simulink model "converterstator"  (Simulink 7.3)
settings: Solver=ode23t  StartTime=0.0  StopTime=.9  RelTol=1e-3
libraries: powerlib x1
settings Model: Creator=lenovo  LastModifiedBy=lenovo

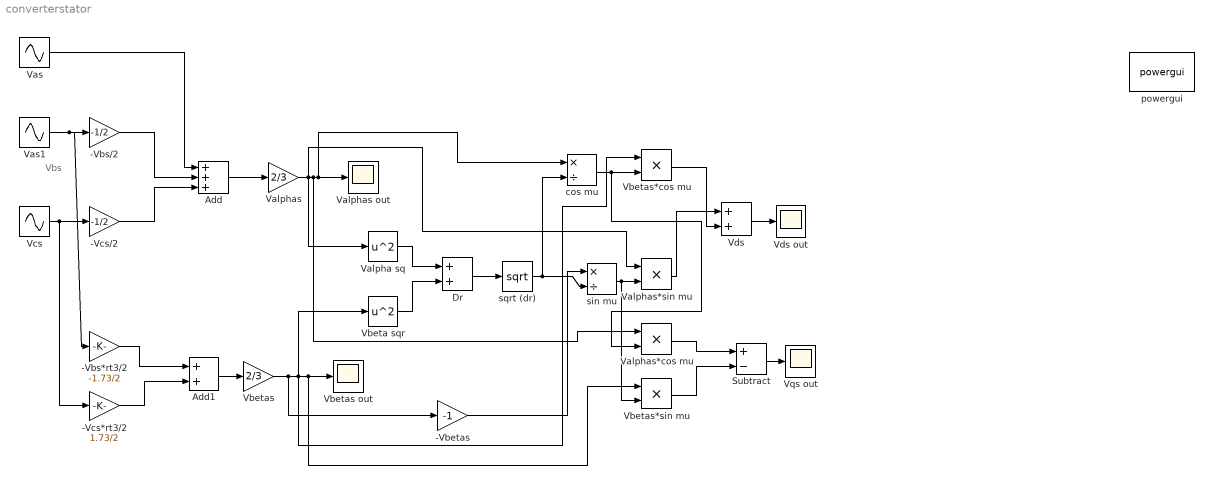
== system converterstator ==
  note: Vbs
  "-Vbetas " : Gain  Gain=-1  ParameterDataType=fixdt(1, 16)  ParameterScaling=2^0  OutDataType=fixdt(1, 16)  OutScaling=2^0
  -Vbs*rt3/2 : Gain  Gain=-1.73/2  ParameterDataType=fixdt(1, 16)  ParameterScaling=2^0  OutDataType=fixdt(1, 16)  OutScaling=2^0
  -Vbs/2 : Gain  Gain=-1/2  ParameterDataType=fixdt(1, 16)  ParameterScaling=2^0  OutDataType=fixdt(1, 16)  OutScaling=2^0
  -Vcs*rt3/2 : Gain  Gain=1.73/2  ParameterDataType=fixdt(1, 16)  ParameterScaling=2^0  OutDataType=fixdt(1, 16)  OutScaling=2^0
  -Vcs/2 : Gain  Gain=-1/2  ParameterDataType=fixdt(1, 16)  ParameterScaling=2^0  OutDataType=fixdt(1, 16)  OutScaling=2^0
  Add : Sum  Inputs=+++  OutDataType=fixdt(1, 16)  OutScaling=2^-10
  Add1 : Sum  OutDataType=fixdt(1, 16)  OutScaling=2^-10
  Dr : Sum  OutDataType=fixdt(1, 16)  OutScaling=2^-10
  Subtract : Sum  Inputs=+-  OutDataType=fixdt(1, 16)  OutScaling=2^-10
  Valpha sq : Math  Operator=square  OutDataType=fixdt(1, 16)  OutScaling=2^0  SaturateOnIntegerOverflow=on
  Valphas : Gain  Gain=2/3  ParameterDataType=fixdt(1, 16)  ParameterScaling=2^0  OutDataType=fixdt(1, 16)  OutScaling=2^0
  Valphas out : Scope
  Valphas*cos mu : Product  OutDataType=fixdt(1, 16)  OutScaling=2^0  RndMeth=Zero
  Valphas*sin mu : Product  OutDataType=fixdt(1, 16)  OutScaling=2^0  RndMeth=Zero
  Vas : Sin  Amplitude=230  Bias=0  Frequency=314  Phase=0  Samples=10  SampleTime=0  Offset=0
  Vas1 : Sin  Amplitude=230  Bias=0  Frequency=314  Phase=-2.09  Samples=10  SampleTime=0  Offset=0
  Vbeta sqr : Math  Operator=square  OutDataType=fixdt(1, 16)  OutScaling=2^0  SaturateOnIntegerOverflow=on
  Vbetas : Gain  Gain=2/3  ParameterDataType=fixdt(1, 16)  ParameterScaling=2^0  OutDataType=fixdt(1, 16)  OutScaling=2^0
  Vbetas out : Scope
  Vbetas*cos mu : Product  OutDataType=fixdt(1, 16)  OutScaling=2^0  RndMeth=Zero
  Vbetas*sin mu : Product  OutDataType=fixdt(1, 16)  OutScaling=2^0  RndMeth=Zero
  Vcs : Sin  Amplitude=230  Bias=0  Frequency=314  Phase=-4.18  Samples=10  SampleTime=0  Offset=0
  Vds : Sum  OutDataType=fixdt(1, 16)  OutScaling=2^-10
  Vds out : Scope
      settings: YMin=-300  YMax=300  SaveName=ScopeData2
  Vqs out : Scope
      settings: YMin=-300  YMax=300  SaveName=ScopeData3
  cos mu : Product  Inputs=*/  OutDataType=fixdt(1, 16)  OutScaling=2^-10
  powergui : powerlib/powergui  Priority=1  SystemSampleTime=-1  SimulationMode=Continuous  SampleTime=50e-6  frequency=60  SPID=off  DisableSnubberDevices=off  DisableRonSwitches=off  DisableVfSwitches=off  SwTol=0  Interpol=off  frequencyindice=60  echomessages=off  HookPort=off  DisplayEquations=off  FunctionMessages=off  EnableUseOfTLC=off  x0status=blocks  RestoreLinks=warning  Frange=[0:2:500]  Ylog=off  Xlog=on  ShowGrid=off  save=off  variable=ZData  ZoomFFT=on  StartTime=0.0  cycles=1  DisplayStyle=1  fundamental=60  FreqAxis=off  MaxFrequency=1000  frequencyindicesteady=1  RmsSteady=1  display=off  Ts=0  methode=off
  sin mu : Product  Inputs=*/  OutDataType=fixdt(1, 16)  OutScaling=2^-10
  sqrt (dr) : Math  Operator=sqrt  OutDataType=fixdt(1, 16)  OutScaling=2^0  SaturateOnIntegerOverflow=on
  wires:
  Vas1/1 -> -Vbs/2/1, -Vbs*rt3/2/1
  Vcs/1 -> -Vcs/2/1, -Vcs*rt3/2/1
  Vas/1 -> Add/1
  -Vbs/2/1 -> Add/2
  -Vcs/2/1 -> Add/3
  Add/1 -> Valphas/1
  -Vbs*rt3/2/1 -> Add1/1
  -Vcs*rt3/2/1 -> Add1/2
  Add1/1 -> Vbetas/1
  Valphas/1 -> Valpha sq/1, Valphas*sin mu/1, Valphas out/1, cos mu/1, Valphas*cos mu/1
  Vbetas/1 -> Vbeta sqr/1, Vbetas*cos mu/1, Vbetas out/1, Vbetas*sin mu/1, "-Vbetas "/1
  Valpha sq/1 -> Dr/1
  Vbeta sqr/1 -> Dr/2
  Dr/1 -> sqrt (dr)/1
  "-Vbetas "/1 -> sin mu/1
  sqrt (dr)/1 -> sin mu/2, cos mu/2
  sin mu/1 -> Valphas*sin mu/2, Vbetas*sin mu/2
  cos mu/1 -> Vbetas*cos mu/2, Valphas*cos mu/2
  Valphas*sin mu/1 -> Vds/1
  Vbetas*cos mu/1 -> Vds/2
  Vds/1 -> Vds out/1
  Valphas*cos mu/1 -> Subtract/1
  Subtract/1 -> Vqs out/1
  Vbetas*sin mu/1 -> Subtract/2
